simulink model "CariPMP"  (R2023b)
settings: Solver=VariableStepAuto  StartTime=0.0  StopTime=10.0  RelTol=1e-3
values from neighbouring files (symbols this model uses):
  A = [0 1 0 0 ... (first row only)    [FindPMP.m]
  B = [B1 B2]    [FindPMP.m]
  C = [0 0 1 0 ... (first row only)    [FindPMP.m]
  P = diag([1, 1])    [FindPMP.m]
  Q = diag([1, 1, 1, 1])    [FindPMP.m]
  R = diag([1, 1])    [FindPMP.m]
settings Model: Creator=izmah  LastModifiedBy=izmah
settings DebuggingCC: UnderSpecifiedDimensionMsg=warning

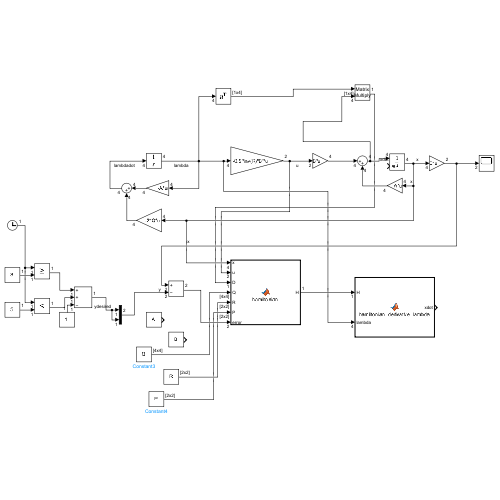
[thumbnail: Simulink's stored preview of the top-level diagram]
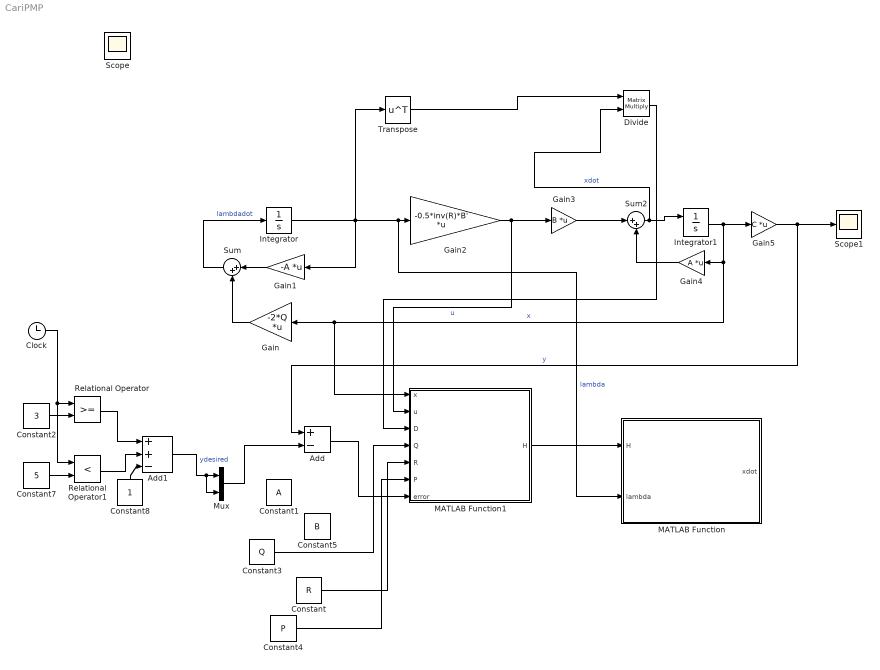
== system CariPMP ==
  Add : Sum  Inputs=+-
  Add1 : Sum  Inputs=++-
  Clock : Clock
  Constant : Constant  Value=R
  Constant1 : Constant  Value=A
  Constant2 : Constant  Value=3
  Constant3 : Constant  Value=Q
  Constant4 : Constant  Value=P
  Constant5 : Constant  Value=B
  Constant7 : Constant  Value=5
  Constant8 : Constant
  Divide : Product  Inputs=**  Multiplication=Matrix(*)
  Gain : Gain  Gain=-2*Q  Multiplication=Matrix(K*u)
  Gain1 : Gain  Gain=-A  Multiplication=Matrix(K*u)
  Gain2 : Gain  Gain=-0.5*inv(R)*B'  Multiplication=Matrix(K*u)
  Gain3 : Gain  Gain=B  Multiplication=Matrix(K*u)
  Gain4 : Gain  Gain=A  Multiplication=Matrix(K*u)
  Gain5 : Gain  Gain=C  Multiplication=Matrix(K*u)
  Integrator : Integrator
  Integrator1 : Integrator  InitialConditionSource=external
  MATLAB Function : MATLAB Function  TreatAsAtomicUnit=on
  MATLAB Function1 : MATLAB Function  TreatAsAtomicUnit=on
  Mux : Mux  Inputs=2
  Relational Operator : RelationalOperator  OutDataTypeStr=boolean  RndMeth=Simplest  InputSameDT=off
  Relational Operator1 : RelationalOperator  Operator=<  OutDataTypeStr=boolean  RndMeth=Simplest  InputSameDT=off
  Scope1 : Scope
  Sum : Sum  Inputs=|++
  Sum2 : Sum  Inputs=|++
  Transpose : Math  Operator=transpose
  Scope : Scope
  wires:
  Gain4/1 -> Sum2/2
  Integrator1/1 -> MATLAB Function1/1(x), Gain/1, Gain4/1, Gain5/1  "x"
  Sum2/1 -> Divide/2, Integrator1/1  "xdot"
  Gain3/1 -> Sum2/1
  Integrator/1 -> MATLAB Function/2(lambda), Gain2/1, Gain1/1, Transpose/1  "lambda"
  Gain1/1 -> Sum/1
  Gain/1 -> Sum/2
  Sum/1 -> Integrator/1  "lambdadot"
  Gain2/1 -> MATLAB Function1/2(u), Gain3/1  "u"
  Gain5/1 -> Scope1/1, Add/1  "y"
  Add1/1 -> Mux/2, Mux/1  "ydesired"
  MATLAB Function1/1(H) -> MATLAB Function/1(H)
  Clock/1 -> Relational Operator/1, Relational Operator1/1
  Constant7/1 -> Relational Operator1/2
  Constant2/1 -> Relational Operator/2
  Relational Operator1/1 -> Add1/2
  Constant8/1 -> Add1/3
  Relational Operator/1 -> Add1/1
  Constant3/1 -> MATLAB Function1/4(Q)
  Constant/1 -> MATLAB Function1/5(R)
  Constant4/1 -> MATLAB Function1/6(P)
  Add/1 -> MATLAB Function1/7(error)
  Mux/1 -> Add/2
  Transpose/1 -> Divide/1
  Divide/1 -> MATLAB Function1/3(D)

== matlab function CariPMP/MATLAB Function1 ==
  data: x input; u input; H output; D input; Q input; R input; P input; error input
function H = hamiltonian(x, u, D, Q, R, P, error)
    % Fungsi untuk menghitung Hamiltonian dengan penalti error output sebagai input
    
    % x - Keadaan saat ini (x(t))
    % u - Kontrol saat ini (u(t))
    % lambda - Costate (lambda(t))
    % A, B - Matriks sistem dinamis
    % Q, R - Matriks biaya untuk keadaan dan kontrol
    % P - Matriks penalti untuk error output
    % error - Error output (y(t) - y_desired) sebagai input
    
    % Fungsi biaya L(x(t), u(t))
    L = x' * Q * x + u' * R * u + error' * P * error;  % Biaya kuadratik untuk keadaan dan kontrol
   
    
    % Hamiltonian H(x(t), u(t), lambda(t), t)
    H = L + D;  % Hamiltonian: biaya + penalti error + costate * dinamika
end

== matlab function CariPMP/MATLAB Function ==
  data: H input; lambda input; xdot output
function xdot = hamiltonian_derivative_lambda(H, lambda)

    xdot = diff(H) / diff(lambda);
end
